simulink model "shower"  (Simulink 10.0)
settings: Solver=ode1  StartTime=0  StopTime=inf  FixedStep=0.12  MaxStep=0.1  RelTol=1e-3  AbsTol=1e-3
PreLoadFcn:
  | fisMatrix=readfis('shower'); k=1;
libraries: fuzblock x1
settings Model: Creator=pascal  LastModifiedBy=bhisma  SimulationMode=external  ExtModeTrigDuration=10000
settings ConfigSet: Description=rtmc9s12target_R2009b
settings SolverCC: AutoScaleAbsTol=off  ZeroCrossControl=DisableAll
settings DataIOCC: SignalLoggingSaveFormat=ModelDataLogs  SaveOutput=off  SaveTime=off  SignalLoggingName=sigsOut
settings OptimizationCC: BlockReduction=off  BooleanDataType=off  ExpressionDepthLimit=2147483647  InitFltsAndDblsToZero=on  LifeSpan=1  EfficientTunableParamExpr=on
settings DebuggingCC: SaveWithParameterizedLinksMsg=none  SignalResolutionControl=TryResolveAllWithWarning  MultiTaskDSMMsg=warning  MultiTaskCondExecSysMsg=none  FcnCallInpInsideContextMsg=warning  StateNameClashWarn=warning
settings HardwareCC: ProdBitPerInt=16  ProdBitPerPointer=16  ProdBitPerSizeT=16  ProdBitPerPtrDiffT=16  ProdEndianess=BigEndian  ProdWordSize=16  ProdHWDeviceType=Motorola HC12
settings SFSimCC: MATLABDynamicMemAlloc=off
settings RTWCC: Description=rtmc9s12-Target for Metrowerks CodeWarrior  SystemTargetFile=mc9s12.tlc  GenerateMakefile=off  TemplateMakefile=mc9s12.tmf
settings CodeAppCC: CustomSymbolStrType=$N$R$M  InternalIdentifier=Classic
settings STFCustomTargetCC: TargetFcnLib=ansi_tfl_tmw.mat  ModelReferenceCompliant=off  IncludeMdlTerminateFcn=off  ERTCustomFileBanners=on  SupportNonInlinedSFcns=off  RemoveResetFunc=on  MATLABClassNameForMDSCustomization=Simulink.SoftwareTarget.ERTCustomization  CPPClassGenCompliant=on  SystemTargetFile=mc9s12.tlc
settings ERTTargetCC: TargetFcnLib=ansi_tfl_tmw.mat  MultiwordLength=2048  ModelReferenceCompliant=off  ParMdlRefBuildCompliant=off  CompOptLevelCompliant=off  ConcurrentExecutionCompliant=off  IncludeMdlTerminateFcn=off  CombineOutputUpdateFcns=off  SupportContinuousTime=on  ModelStepFunctionPrototypeControlCompliant=off  GRTInterface=on  UseToolchainInfoCompliant=off  ExtModeMexFile=ext_serial_mc9s12_comm  ExtModeMexArgs=1,2,115200  ERTCustomFileTemplate=mc9s12_file_process.tlc  ConvertIfToSwitch=off  SuppressUnreachableDefaultCases=off
settings CustomProperty: DataType=RTWOptions_EnumType_C__Users_fw__SVN_rtmc9s12-target_trunk_rtmc9s12_CW_R2009b_bin_mc9s12_1mc9s12_TargetBoard  Value=Dragon12Plus
settings EnumStrPairs: String=Dragon12
settings ConfigComp: CovExternalEMLEnable=off

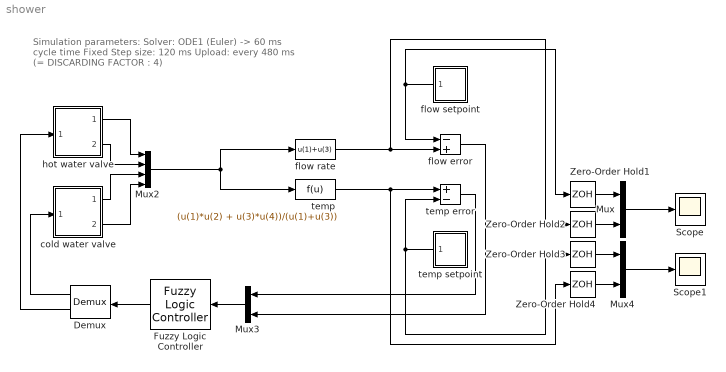
== system shower ==
  note: Simulation parameters:
      | Solver: ODE1 (Euler)  ->  60 ms cycle time
      | Fixed Step size: 120 ms
      | Upload: every 480 ms   (= DISCARDING FACTOR : 4)
  Demux : Demux  Outputs=2
  Fuzzy Logic Controller : fuzblock/Fuzzy Logic  Controller  SystemSampleTime=-1  fis=fisMatrix
  Mux : Mux  Inputs=2
  Mux2 : Mux
  Mux3 : Mux  Inputs=2
  Mux4 : Mux  Inputs=2
  Scope : Scope
  Scope1 : Scope
  Zero-Order Hold{1..4} (4 alike) : ZeroOrderHold  SampleTime=0.48
  cold water valve : Subsystem
  flow error : Sum  Inputs=-+  SaturateOnIntegerOverflow=on  InputSameDT=on  OutDataTypeStr=Inherit: Same as first input
  flow setpoint : Subsystem
  flow rate : Fcn  Expr=u(1)+u(3)
  hot water valve : Subsystem
  temp : Fcn  Expr=(u(1)*u(2) + u(3)*u(4))/(u(1)+u(3))
  temp error : Sum  Inputs=+-  SaturateOnIntegerOverflow=on  InputSameDT=on  OutDataTypeStr=Inherit: Same as first input
  temp setpoint : Subsystem
  wires:
  cold water valve/1(out_1) -> Mux2/3
  hot water valve/1(out_1) -> Mux2/1
  hot water valve/2(out_2) -> Mux2/2
  cold water valve/2(out_2) -> Mux2/4
  Demux/1 -> cold water valve/1(in_1)
  Demux/2 -> hot water valve/1(in_1)
  Mux3/1 -> Fuzzy Logic Controller/1
  temp error/1 -> Mux3/1
  flow error/1 -> Mux3/2
  Fuzzy Logic Controller/1 -> Demux/1
  Mux2/1 -> flow rate/1, temp/1
  temp/1 -> temp error/1, Zero-Order Hold4/1
  temp setpoint/1(out_1) -> temp error/2, Zero-Order Hold3/1
  flow rate/1 -> flow error/2, Zero-Order Hold2/1
  flow setpoint/1(out_1) -> flow error/1, Zero-Order Hold1/1
  Zero-Order Hold1/1 -> Mux/1
  Zero-Order Hold2/1 -> Mux/2
  Zero-Order Hold3/1 -> Mux4/1
  Zero-Order Hold4/1 -> Mux4/2
  Mux/1 -> Scope/1
  Mux4/1 -> Scope1/1

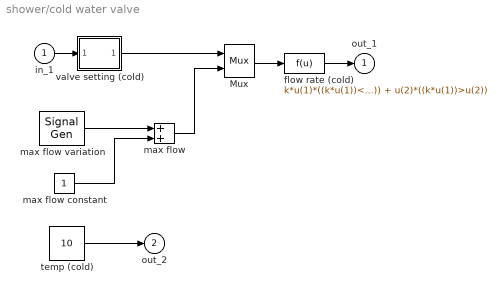
== system shower/cold water valve ==
  in_1 : Inport
  Mux : Mux  Inputs=2
  flow rate (cold) : Fcn  Expr=k*u(1)*((k*u(1))<=u(2)) + u(2)*((k*u(1))>u(2))
  max flow : Sum  SaturateOnIntegerOverflow=on  InputSameDT=on  OutDataTypeStr=Inherit: Same as first input
  max flow constant : Constant
  max flow variation : SignalGenerator  Amplitude=0.000000  Frequency=0.101325  Units=rad/sec
  temp (cold) : Constant  Value=10
  valve setting (cold) : Subsystem  mask(Limited Integrator.){lower_limit=0.001, upper_limit=2, X0=0.1}
      mask prompts: lower_limit "Lower bound:"; upper_limit "Upper bound:"; X0 "Initial condition:"
      mask help: Limited Integrator
      mask Help: Implements a limited integrator with \nan expression of the form:\n\nif(x<=lb and u<0) or (x>=ub and u>0)\n   xdot=0\nelse\n   xdot=u
      mask Display: plot(-1,-0.2,3.5,1.2,[0.05,1,2,2.9],[0,0,1,1]);disp(' 1/s    ')
  out_1 : Outport  InitialOutput=0
  out_2 : Outport  Port=2  InitialOutput=0
  wires:
  max flow/1 -> Mux/2
  max flow variation/1 -> max flow/1
  max flow constant/1 -> max flow/2
  temp (cold)/1 -> out_2/1
  flow rate (cold)/1 -> out_1/1
  in_1/1 -> valve setting (cold)/1(Inport)
  Mux/1 -> flow rate (cold)/1
  valve setting (cold)/1(Outport) -> Mux/1

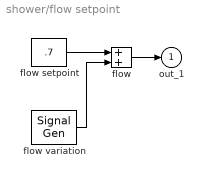
== system shower/flow setpoint ==
  flow : Sum  SaturateOnIntegerOverflow=on  InputSameDT=on  OutDataTypeStr=Inherit: Same as first input
  flow setpoint : Constant  Value=.7
  flow variation : SignalGenerator  WaveForm=square  Amplitude=0.200000  Frequency=0.300000  Units=rad/sec
  out_1 : Outport  InitialOutput=0
  wires:
  flow setpoint/1 -> flow/1
  flow variation/1 -> flow/2
  flow/1 -> out_1/1

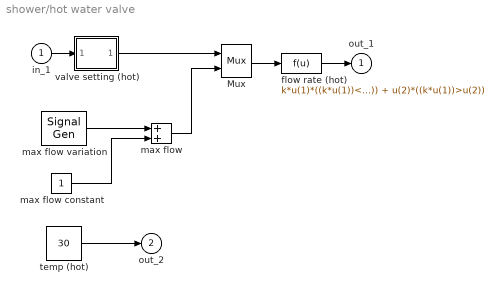
== system shower/hot water valve ==
  in_1 : Inport
  Mux : Mux  Inputs=2
  flow rate (hot) : Fcn  Expr=k*u(1)*((k*u(1))<=u(2)) + u(2)*((k*u(1))>u(2))
  max flow : Sum  SaturateOnIntegerOverflow=on  InputSameDT=on  OutDataTypeStr=Inherit: Same as first input
  max flow constant : Constant
  max flow variation : SignalGenerator  Amplitude=0.000000  Frequency=0.300000  Units=rad/sec
  temp (hot) : Constant  Value=30
  valve setting (hot) : Subsystem  mask(Limited Integrator.){lower_limit=0.001, upper_limit=2, X0=.1}
      mask prompts: lower_limit "Lower bound:"; upper_limit "Upper bound:"; X0 "Initial condition:"
      mask help: Limited Integrator
      mask Help: Implements a limited integrator with \nan expression of the form:\n\nif(x<=lb and u<0) or (x>=ub and u>0)\n   xdot=0\nelse\n   xdot=u
      mask Display: plot(-1,-0.2,3.5,1.2,[0.05,1,2,2.9],[0,0,1,1]);disp(' 1/s    ')
  out_1 : Outport  InitialOutput=0
  out_2 : Outport  Port=2  InitialOutput=0
  wires:
  valve setting (hot)/1(Outport) -> Mux/1
  Mux/1 -> flow rate (hot)/1
  in_1/1 -> valve setting (hot)/1(Inport)
  flow rate (hot)/1 -> out_1/1
  temp (hot)/1 -> out_2/1
  max flow constant/1 -> max flow/2
  max flow variation/1 -> max flow/1
  max flow/1 -> Mux/2

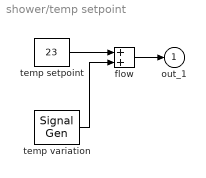
== system shower/temp setpoint ==
  flow : Sum  SaturateOnIntegerOverflow=on  InputSameDT=on  OutDataTypeStr=Inherit: Same as first input
  temp setpoint : Constant  Value=23
  temp variation : SignalGenerator  WaveForm=square  Amplitude=4.000000  Frequency=0.214320  Units=rad/sec
  out_1 : Outport  InitialOutput=0
  wires:
  flow/1 -> out_1/1
  temp variation/1 -> flow/2
  temp setpoint/1 -> flow/1

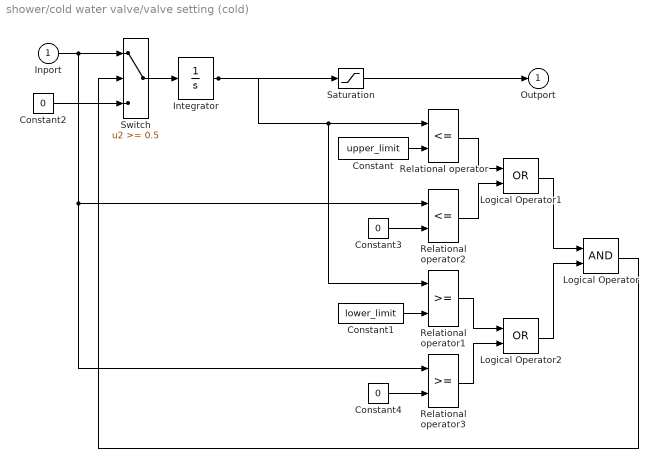
== system shower/cold water valve/valve setting (cold) ==
  Inport : Inport
  Constant : Constant  Value=upper_limit
  Constant1 : Constant  Value=lower_limit
  Constant2 : Constant  Value=0
  Constant3 : Constant  Value=0
  Constant4 : Constant  Value=0
  Integrator : Integrator  InitialCondition=X0
  Logical Operator : Logic
  Logical Operator1 : Logic  Operator=OR
  Logical Operator2 : Logic  Operator=OR
  Relational operator : RelationalOperator  Operator=<=  RndMeth=Nearest  InputSameDT=on
  Relational operator1 : RelationalOperator  RndMeth=Nearest  InputSameDT=on
  Relational operator2 : RelationalOperator  Operator=<=  RndMeth=Nearest  InputSameDT=on
  Relational operator3 : RelationalOperator  RndMeth=Nearest  InputSameDT=on
  Saturation : Saturate  UpperLimit=upper_limit  LowerLimit=lower_limit
  Switch : Switch  Threshold=0.5  SaturateOnIntegerOverflow=on  InputSameDT=on
  Outport : Outport  InitialOutput=0
  wires:
  Constant4/1 -> Relational operator3/2
  Constant3/1 -> Relational operator2/2
  Logical Operator2/1 -> Logical Operator/2
  Relational operator3/1 -> Logical Operator2/2
  Relational operator1/1 -> Logical Operator2/1
  Logical Operator1/1 -> Logical Operator/1
  Relational operator2/1 -> Logical Operator1/2
  Relational operator/1 -> Logical Operator1/1
  Constant2/1 -> Switch/3
  Logical Operator/1 -> Switch/2
  Constant1/1 -> Relational operator1/2
  Constant/1 -> Relational operator/2
  Switch/1 -> Integrator/1
  Inport/1 -> Switch/1, Relational operator2/1, Relational operator3/1
  Integrator/1 -> Relational operator1/1, Relational operator/1, Saturation/1
  Saturation/1 -> Outport/1

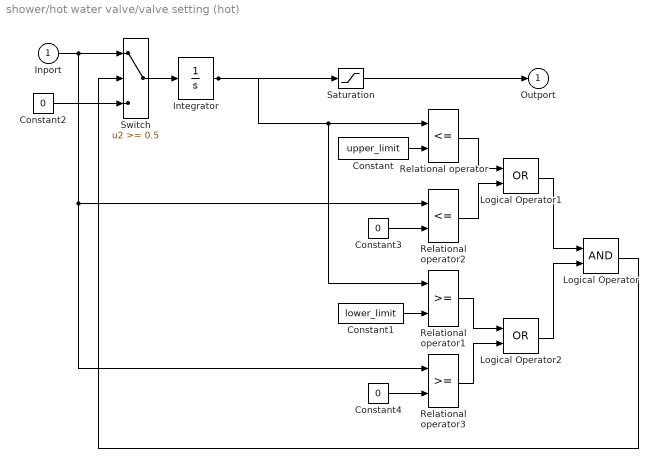
== system shower/hot water valve/valve setting (hot) ==
  Inport : Inport
  Constant : Constant  Value=upper_limit
  Constant1 : Constant  Value=lower_limit
  Constant2 : Constant  Value=0
  Constant3 : Constant  Value=0
  Constant4 : Constant  Value=0
  Integrator : Integrator  InitialCondition=X0
  Logical Operator : Logic
  Logical Operator1 : Logic  Operator=OR
  Logical Operator2 : Logic  Operator=OR
  Relational operator : RelationalOperator  Operator=<=  RndMeth=Nearest  InputSameDT=on
  Relational operator1 : RelationalOperator  RndMeth=Nearest  InputSameDT=on
  Relational operator2 : RelationalOperator  Operator=<=  RndMeth=Nearest  InputSameDT=on
  Relational operator3 : RelationalOperator  RndMeth=Nearest  InputSameDT=on
  Saturation : Saturate  UpperLimit=upper_limit  LowerLimit=lower_limit
  Switch : Switch  Threshold=0.5  SaturateOnIntegerOverflow=on  InputSameDT=on
  Outport : Outport  InitialOutput=0
  wires:
  Saturation/1 -> Outport/1
  Inport/1 -> Switch/1, Relational operator2/1, Relational operator3/1
  Switch/1 -> Integrator/1
  Constant/1 -> Relational operator/2
  Constant1/1 -> Relational operator1/2
  Logical Operator/1 -> Switch/2
  Constant2/1 -> Switch/3
  Relational operator/1 -> Logical Operator1/1
  Relational operator2/1 -> Logical Operator1/2
  Logical Operator1/1 -> Logical Operator/1
  Relational operator1/1 -> Logical Operator2/1
  Relational operator3/1 -> Logical Operator2/2
  Logical Operator2/1 -> Logical Operator/2
  Constant3/1 -> Relational operator2/2
  Constant4/1 -> Relational operator3/2
  Integrator/1 -> Saturation/1, Relational operator1/1, Relational operator/1
